simulink model "HVDC_Case_B"  (R2024b)
settings: Solver=VariableStepAuto  StartTime=0.0  StopTime=5  RelTol=1e-3
undefined symbols (not defined in the file): D11, Delta, leading, pulse
libraries: spsUniversalBridgeLib x4, spsSeriesRLCBranchLib x3, spsPLL3phLib x2, spsPower3phInstantaneousLib x2, spsPulseGeneratorThyristor12PulseLib x2, spsThreePhaseTransformerThreeWindingsLib x2, spsThreePhaseVIMeasurementLib x2, spsThreePhaseSourceLib x2, spsVoltageMeasurementLib x2, spsMeanLib x1, slpidlib x1, simulink x1
settings Model: Creator=Eng.Abd-Elrhman Saad  LastModifiedBy=Eng.Abd-Elrhman Saad

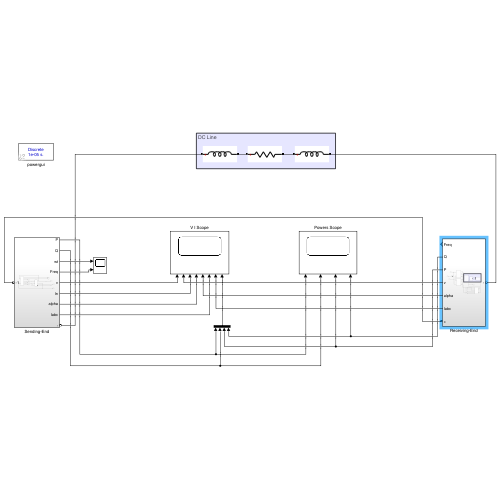
[thumbnail: Simulink's stored preview of the top-level diagram]
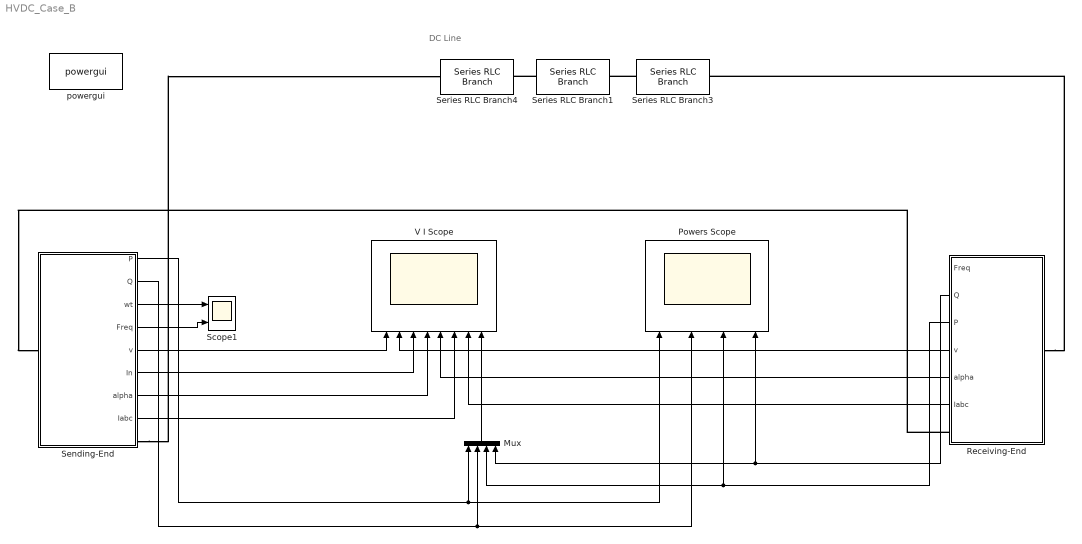
== system HVDC_Case_B ==
  note: DC Line
  Mux : Mux
  Powers Scope : Scope  NumInputPorts=4
  Receiving-End : Subsystem
  Scope1 : Scope  NumInputPorts=2
  Sending-End : Subsystem
  Series RLC Branch1 : spsSeriesRLCBranchLib/Series RLC Branch  LConnTagsString=__new0  RConnTagsString=__new0  BranchType=R  Resistance=5  Inductance=1e-3  SetiL0=off  InitialCurrent=0  Capacitance=1e-6  Setx0=off  InitialVoltage=0  Measurements=None
  Series RLC Branch3 : spsSeriesRLCBranchLib/Series RLC Branch  LConnTagsString=__new0  RConnTagsString=__new0  BranchType=L  Resistance=5  Inductance=0.3  SetiL0=off  InitialCurrent=1e5  Capacitance=1e-6  Setx0=off  InitialVoltage=0  Measurements=None
  Series RLC Branch4 : spsSeriesRLCBranchLib/Series RLC Branch  LConnTagsString=__new0  RConnTagsString=__new0  BranchType=L  Resistance=5  Inductance=0.3  SetiL0=off  InitialCurrent=1e5  Capacitance=1e-6  Setx0=off  InitialVoltage=0  Measurements=None
  V I Scope : Scope  NumInputPorts=8
  powergui : sps_lib/powergui  Priority=1  SimulationMode=Discrete  SampleTime=1e-5  frequency=60  Iterations=50  frequencyindice=50  Pbase=100e6  ErrMax=1e-4  UnitsV=kV  UnitsW=MW  buscounter=0  FunctionMessages=off  echomessages=off  EnableUseOfTLC=off  CurrentSourceSwitches=off  DisableSnubberDevices=off  DisableRonSwitches=off  DisableVfSwitches=off  DisplayEquations=off  AutomaticDiscreteSolvers=off  SolverType=Tustin/Backward Euler (TBE)  Interpol=off  ExternalGateDelay=off  methode=off  Ts=100  x0status=blocks  SPID=on  SwTol=0  HookPort=off  NonlinearTolerance=1e-4  nMaxIteration=100  ContinueOnMaxIteration=off  RestoreLinks=warning  ResistiveCurrentMeasurement=off  Frange=[0:2:500]  Ylog=off  Xlog=on  ShowGrid=off  save=off  variable=ZData  structure=0  ZoomFFT=off  StartTime=0.0  cycles=1  DisplayStyle=1  fundamental=60  FreqAxis=off  MaxFrequency=1000  frequencyindicesteady=1  RmsSteady=1  display=off
  wires:
  Mux/1 -> V I Scope/8
  Sending-End/2(Q) -> Powers Scope/2, Mux/2
  Sending-End/1(P) -> Mux/1, Powers Scope/1
  Sending-End/3(wt) -> Scope1/1
  Sending-End/4(Freq) -> Scope1/2
  Sending-End/5(v) -> V I Scope/1
  Sending-End/6(In) -> V I Scope/3
  Sending-End/7(alpha) -> V I Scope/4
  Sending-End/8(Iabc) -> V I Scope/6
  Receiving-End/2(Q) -> Mux/4, Powers Scope/4
  Receiving-End/3(P) -> Mux/3, Powers Scope/3
  Receiving-End/4(v) -> V I Scope/2
  Receiving-End/5(alpha) -> V I Scope/5
  Receiving-End/6(Iabc) -> V I Scope/7
  connections:
  Receiving-End/RConn1 -- Sending-End/LConn1
  Receiving-End/LConn1 -- Series RLC Branch3/RConn1
  Series RLC Branch1/LConn1 -- Series RLC Branch4/RConn1
  Sending-End/RConn1 -- Series RLC Branch4/LConn1
  Series RLC Branch3/LConn1 -- Series RLC Branch1/RConn1

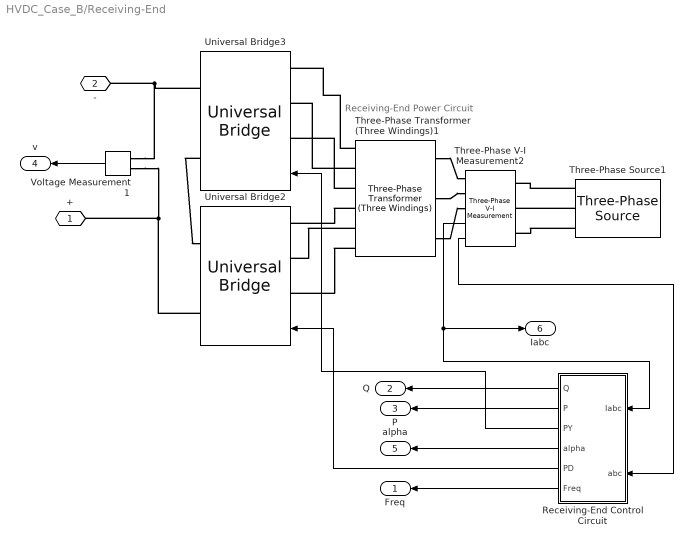
== system HVDC_Case_B/Receiving-End ==
  note: Receiving-End Power Circuit
  Receiving-End Control Circuit : Subsystem
  Three-Phase Transformer (Three Windings)1 : spsThreePhaseTransformerThreeWindingsLib/Three-Phase Transformer (Three Windings)  Winding1Connection=Yg  Winding2Connection=Delta (D11)  Winding3Connection=Y  CoreType=Three single-phase transformers  SetSaturation=off  Hysteresis=off  DataFile='hysteresis'  SetInitialFlux=off  Measurements=None  UNITS=pu  NominalPower=[ 2e9 , 50 ]  Winding1=[ 77.618e3 , 0.002 , 1e-6 ]  Winding2=[ 77.618e3 , 0.002 , 1e-6 ]  Winding3=[ 77.618e3 , 0.002 , 1e-6 ]  Rm=1e6  Lm=1e6  L0=1169.8  Saturation=[ 0,0 ; 0.0024,1.2 ; 1.0,1.52 ]  InitialFluxes=[1528.2 -1528.2 1337.2]  BreakLoop=off  DiscreteSolver=Trapezoidal iterative  DataType=off  TransfoNumber=1
      settings: LibrarySourceBlock=|
      | sps_lib/Power Grid Elements/Three-Phase
      | Transformer
      | (Three Windings)
  Three-Phase V-I Measurement2 : spsThreePhaseVIMeasurementLib/Three-Phase V-I Measurement  VoltageMeasurement=phase-to-ground  SetLabelV=off  LabelV=Vabc  Vpu=off  VpuLL=off  CurrentMeasurement=yes  SetLabelI=off  LabelI=Iabc  Ipu=off  Pbase=100e6  Vbase=500e3  OutputType=Complex  PhasorSimulation=off  PSBequivalent=0
  Three-Phase Source1 : spsThreePhaseSourceLib/Three-Phase Source  InternalConnection=Yg  VoltagePhases=off  Voltage=77.618e3  PhaseAngle=0  Voltage_phases=[25e3 25e3 25e3]/sqrt(3)  PhaseAngles_phases=[0 -120 +120]  Frequency=50  NonIdealSource=off  SpecifyImpedance=off  Resistance=0.8929  Inductance=16.58e-3  ShortCircuitLevel=100e6  BaseVoltage=25e3  XRratio=7  BusType=swing  Pref=10e3  Qref=0  Prefabc=[10e3, 10e3, 10e3]  Qrefabc=[0, 0, 0]  Qmin=-inf  Qmax=inf
  Universal Bridge2 : spsUniversalBridgeLib/Universal Bridge  Arms=3  SnubberResistance=1e5  SnubberCapacitance=inf  Device=Thyristors  Ron=1e-3  Lon=0  ForwardVoltages="[  0  0  ]"  ForwardVoltage=0  GTOparameters=[ 10e-6 , 20e-6 ]  IGBTparameters=[ 1e-6 , 2e-6 ]  Measurements=None  Measurements_2=None  converterType=Rectifier
  Universal Bridge3 : spsUniversalBridgeLib/Universal Bridge  Arms=3  SnubberResistance=1e5  SnubberCapacitance=inf  Device=Thyristors  Ron=1e-3  Lon=0  ForwardVoltages="[  0  0  ]"  ForwardVoltage=0  GTOparameters=[ 10e-6 , 20e-6 ]  IGBTparameters=[ 1e-6 , 2e-6 ]  Measurements=None  Measurements_2=None  converterType=Rectifier
  Voltage Measurement1 : spsVoltageMeasurementLib/Voltage Measurement  PhasorSimulation=off  OutputType=Complex  PSBequivalent=0
  + : PMIOPort  Side=Right
  - : PMIOPort  Port=2  Side=Left
  Freq : Outport
  Q : Outport  Port=2
  P : Outport  Port=3
  v : Outport  Port=4
  alpha : Outport  Port=5
  Iabc : Outport  Port=6
  wires:
  Receiving-End Control Circuit/3(PY) -> Universal Bridge3/1
  Receiving-End Control Circuit/5(PD) -> Universal Bridge2/1
  Three-Phase V-I Measurement2/1 -> Receiving-End Control Circuit/2(abc)
  Three-Phase V-I Measurement2/2 -> Receiving-End Control Circuit/1(Iabc), Iabc/1
  Receiving-End Control Circuit/2(P) -> P/1
  Receiving-End Control Circuit/1(Q) -> Q/1
  Voltage Measurement1/1 -> v/1
  Receiving-End Control Circuit/4(alpha) -> alpha/1
  Receiving-End Control Circuit/6(Freq) -> Freq/1
  connections:
  Voltage Measurement1/LConn1 -- -/RConn1 -- Universal Bridge3/RConn2
  Universal Bridge3/RConn1 -- Universal Bridge2/RConn2
  Voltage Measurement1/LConn2 -- Universal Bridge2/RConn1 -- +/RConn1
  Three-Phase Transformer (Three Windings)1/LConn1 -- Three-Phase V-I Measurement2/RConn1
  Three-Phase Source1/RConn3 -- Three-Phase V-I Measurement2/LConn3
  Three-Phase Source1/RConn2 -- Three-Phase V-I Measurement2/LConn2
  Three-Phase Source1/RConn1 -- Three-Phase V-I Measurement2/LConn1
  Three-Phase Transformer (Three Windings)1/LConn2 -- Three-Phase V-I Measurement2/RConn2
  Three-Phase Transformer (Three Windings)1/LConn3 -- Three-Phase V-I Measurement2/RConn3
  Three-Phase Transformer (Three Windings)1/RConn1 -- Universal Bridge2/LConn1
  Three-Phase Transformer (Three Windings)1/RConn2 -- Universal Bridge2/LConn2
  Three-Phase Transformer (Three Windings)1/RConn3 -- Universal Bridge2/LConn3
  Three-Phase Transformer (Three Windings)1/RConn4 -- Universal Bridge3/LConn1
  Three-Phase Transformer (Three Windings)1/RConn5 -- Universal Bridge3/LConn2
  Three-Phase Transformer (Three Windings)1/RConn6 -- Universal Bridge3/LConn3

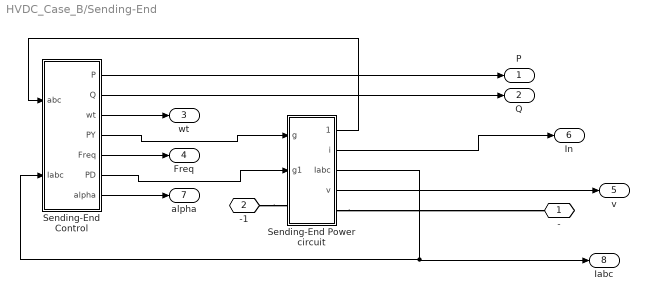
== system HVDC_Case_B/Sending-End ==
  Sending-End Control : Subsystem
  Sending-End Power circuit : Subsystem
  - : PMIOPort  Side=Right
  -1 : PMIOPort  Port=2  Side=Left
  P : Outport
  Q : Outport  Port=2
  wt : Outport  Port=3
  Freq : Outport  Port=4
  v : Outport  Port=5
  In : Outport  Port=6
  alpha : Outport  Port=7
  Iabc : Outport  Port=8
  wires:
  Sending-End Power circuit/3(Iabc) -> Iabc/1, Sending-End Control/2(Iabc)
  Sending-End Power circuit/1(Vabc) -> Sending-End Control/1(abc)
  Sending-End Power circuit/2(i) -> In/1
  Sending-End Control/6(PD) -> Sending-End Power circuit/2(g1)
  Sending-End Control/4(PY) -> Sending-End Power circuit/1(g)
  Sending-End Control/2(Q) -> Q/1
  Sending-End Power circuit/4(v) -> v/1
  Sending-End Control/5(Freq) -> Freq/1
  Sending-End Control/7(alpha) -> alpha/1
  Sending-End Control/3(wt) -> wt/1
  Sending-End Control/1(P) -> P/1
  connections:
  -1/RConn1 -- Sending-End Power circuit/LConn1
  Sending-End Power circuit/RConn1 -- -/RConn1

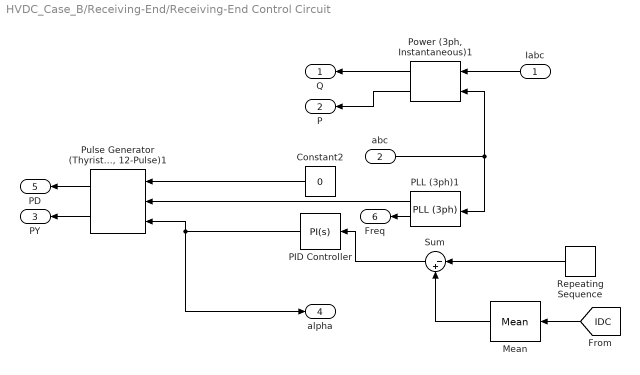
== system HVDC_Case_B/Receiving-End/Receiving-End Control Circuit ==
  Iabc : Inport
  abc : Inport  Port=2
  Constant2 : Constant  Value=0
  Mean : spsMeanLib/Mean  Freq=50  Vinit=0  Ts=0
  PID Controller : slpidlib/PID Controller  Controller=PI  Form=Parallel  TimeDomain=Continuous-time  UseExternalTs=off  SampleTime=-1  IntegratorMethod=Forward Euler  FilterMethod=Forward Euler  ControllerParametersSource=internal  P=0.003  I=0.05  UseKiTs=off  D=0  UseExternalDerivativeSource=off  N=100  UseFilter=on  TunerSelectOption=Transfer Function Based (PID Tuner App)  InitialConditionSource=internal  InitialConditionForIntegrator=110  InitialConditionForFilter=0  DifferentiatorICPrevScaledInput=0  ExternalReset=none  TrackingMode=off  Kt=1  LimitOutput=on  SatLimitsSource=internal  UpperSaturationLimit=160  LowerSaturationLimit=100  LinearizeAsGain=on  AntiWindupMode=none  Kb=1  LimitIntegrator=off  UpperIntegratorSaturationLimit=inf  LowerIntegratorSaturationLimit=-inf  POutMin=[]  POutMax=[]  IOutMin=[]  IOutMax=[]  DOutMin=[]  DOutMax=[]  NOutMin=[]  NOutMax=[]  SumOutMin=[]  SumOutMax=[]  SaturationOutMin=[]  SaturationOutMax=[]  PParamMin=[]  PParamMax=[]  IParamMin=[]  IParamMax=[]  DParamMin=[]  DParamMax=[]  NParamMin=[]  NParamMax=[]  KbParamMin=[]  KbParamMax=[]  KtParamMin=[]  KtParamMax=[]  KbOutMin=[]  KbOutMax=[]  KtOutMin=[]  KtOutMax=[]  IntegratorOutMin=[]  IntegratorOutMax=[]  FilterOutMin=[]  FilterOutMax=[]  SumI1OutMin=[]  SumI1OutMax=[]  SumI2OutMin=[]  SumI2OutMax=[]  SumI3OutMin=[]  SumI3OutMax=[]  SumI4OutMin=[]  SumI4OutMax=[]  SumDOutMin=[]  SumDOutMax=[]  DifferentiatorOutMin=[]  DifferentiatorOutMax=[]  FilterDiffOutCoefMin=[]  FilterDiffOutCoefMax=[]  ReciprocalOutMin=[]  ReciprocalOutMax=[]  SumDenOutMin=[]  SumDenOutMax=[]  SumNumOutMin=[]  SumNumOutMax=[]  DivideOutMin=[]  DivideOutMax=[]  UdiffTsProdOutMin=[]  UdiffTsProdOutMax=[]  NTsProdOutMin=[]  NTsProdOutMax=[]  UintegralTsProdOutMin=[]  UintegralTsProdOutMax=[]  UngainTsProdOutMin=[]  UngainTsProdOutMax=[]  ClampingZeroOutDataTypeStr=Inherit: Inherit via back propagation  ClampingZeroOutMin=[]  ClampingZeroOutMax=[]  FilterDenConstantOutDataTypeStr=Inherit: Inherit via back propagation  FilterDenConstantOutMin=[]  FilterDenConstantOutMax=[]  PCopyOutDataTypeStr=Inherit: Inherit via back propagation  PCopyOutMin=[]  PCopyOutMax=[]  NCopyOutDataTypeStr=Inherit: Inherit via back propagation  NCopyOutMin=[]  NCopyOutMax=[]  IntegratorContinuousStateAttributes=''  IntegratorStateMustResolveToSignalObject=off  IntegratorRTWStateStorageClass=Auto  FilterContinuousStateAttributes=''  FilterStateMustResolveToSignalObject=off  FilterRTWStateStorageClass=Auto  ParallelPVariant=InternalParameters  IdealPVariant=Disabled  IVariant=InternalParameters  DVariant=Disabled  IntegratorVariant=Continuous  SatVariant=Enabled  AWVariant=Passthrough  PCopyVariant=Disabled  TRVariant=Disabled  FdbkBlocksVariant=Forward  IdealPFdbkVariant=Disabled  SatFdbkVariant=Disabled  DerivativeFilterVariant=Disabled  NVariant=Disabled  NCopyVariant=Disabled_SignalSpec  FilterICVariant=Disabled  IntegratorICVariant=InternalICs  ExternalResetVariant=Disabled  TRSumVariant=Passthrough  SumFdbkVariant=Disabled  SumVariant=Sum_PI  TsampFilterVariant=InternalTs  TsampNgainVariant=Passthrough  TsampIntegralVariant=Disabled_SignalSpec  ExternalSaturationOutDataTypeStr=Inherit: Same as second input  DerivativeSourceVariant=Disabled  PreIntVariant=InternalPreInt
  PLL (3ph)1 : spsPLL3phLib/PLL (3ph)  Fmin=45  Par_Init=[0, 50]  ParK=[180, 3200, 1]  TcD=1e-4  MaxRateChangeFreq=12  FilterCutOffFreq=25  Ts=0  AGC=on
  "Power (3ph, Instantaneous)1" : spsPower3phInstantaneousLib/Power (3ph, Instantaneous)
  "Pulse Generator (Thyristor, 12-Pulse)1" : spsPulseGeneratorThyristor12PulseLib/Pulse Generator (Thyristor, 12-Pulse)  GenType=12-pulse  Delta=D11 (leading)  pwidth=30  Double_Pulse=off  Ts=0
      settings: LibrarySourceBlock=|
      | sps_lib/Power Electronics/Power Electronics Control/Pulse Generator
      | (Thyristor, 12-Pulse)
  Repeating Sequence : simulink/Sources/Repeating Sequence  rep_seq_t=[0, 0.2, 2, 2.0001, 4, 4.0001, 10]  rep_seq_y=[0, 6650, 6650, 5700, 5700, 6650, 6650]
  Sum : Sum  Inputs=|-+
  Q : Outport
  P : Outport  Port=2
  PY : Outport  Port=3
  alpha : Outport  Port=4
  PD : Outport  Port=5
  Freq : Outport  Port=6
  wires:
  Constant2/1 -> "Pulse Generator (Thyristor, 12-Pulse)1"/3
  abc/1 -> "Power (3ph, Instantaneous)1"/1, PLL (3ph)1/1
  PLL (3ph)1/2 -> "Pulse Generator (Thyristor, 12-Pulse)1"/2
  "Power (3ph, Instantaneous)1"/2 -> Q/1
  PID Controller/1 -> alpha/1, "Pulse Generator (Thyristor, 12-Pulse)1"/1
  "Pulse Generator (Thyristor, 12-Pulse)1"/2 -> PD/1
  PLL (3ph)1/1 -> Freq/1
  "Pulse Generator (Thyristor, 12-Pulse)1"/1 -> PY/1
  Iabc/1 -> "Power (3ph, Instantaneous)1"/2
  "Power (3ph, Instantaneous)1"/1 -> P/1
  Sum/1 -> PID Controller/1
  Mean/1 -> Sum/2
  Repeating Sequence/1 -> Sum/1
  [IDC] -> Mean/1

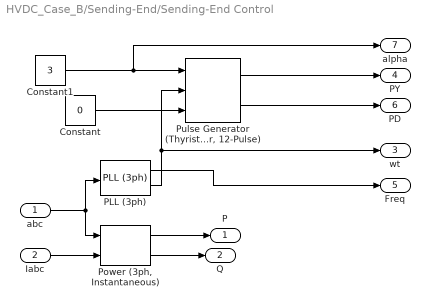
== system HVDC_Case_B/Sending-End/Sending-End Control ==
  abc : Inport
  Iabc : Inport  Port=2
  Constant : Constant  Value=0
  Constant1 : Constant  Value=3
  PLL (3ph) : spsPLL3phLib/PLL (3ph)  Fmin=45  Par_Init=[0, 50]  ParK=[180, 3200, 1]  TcD=1e-4  MaxRateChangeFreq=12  FilterCutOffFreq=25  Ts=0  AGC=on
  "Power (3ph, Instantaneous)" : spsPower3phInstantaneousLib/Power (3ph, Instantaneous)
  "Pulse Generator (Thyristor, 12-Pulse)" : spsPulseGeneratorThyristor12PulseLib/Pulse Generator (Thyristor, 12-Pulse)  GenType=12-pulse  Delta=D11 (leading)  pwidth=30  Double_Pulse=off  Ts=0
      settings: LibrarySourceBlock=|
      | sps_lib/Power Electronics/Power Electronics Control/Pulse Generator
      | (Thyristor, 12-Pulse)
  P : Outport
  Q : Outport  Port=2
  wt : Outport  Port=3
  PY : Outport  Port=4
  Freq : Outport  Port=5
  PD : Outport  Port=6
  alpha : Outport  Port=7
  wires:
  PLL (3ph)/2 -> "Pulse Generator (Thyristor, 12-Pulse)"/2, wt/1
  Constant1/1 -> alpha/1, "Pulse Generator (Thyristor, 12-Pulse)"/1
  Iabc/1 -> "Power (3ph, Instantaneous)"/2
  Constant/1 -> "Pulse Generator (Thyristor, 12-Pulse)"/3
  abc/1 -> "Power (3ph, Instantaneous)"/1, PLL (3ph)/1
  "Power (3ph, Instantaneous)"/1 -> P/1
  "Pulse Generator (Thyristor, 12-Pulse)"/2 -> PD/1
  "Power (3ph, Instantaneous)"/2 -> Q/1
  "Pulse Generator (Thyristor, 12-Pulse)"/1 -> PY/1
  PLL (3ph)/1 -> Freq/1

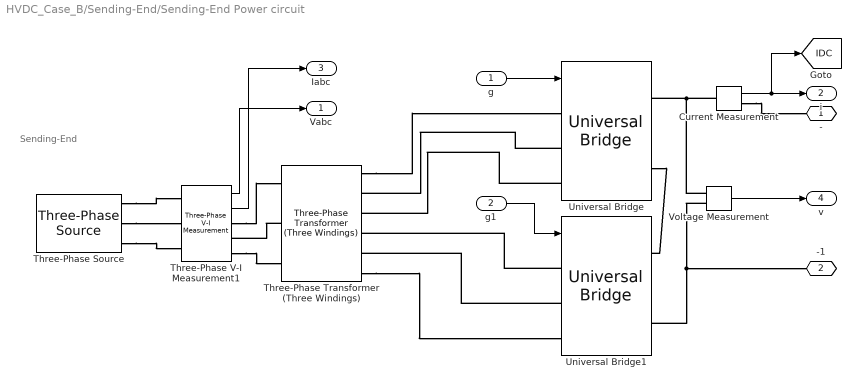
== system HVDC_Case_B/Sending-End/Sending-End Power circuit ==
  note: Sending-End
  g : Inport
  g1 : Inport  Port=2
  Current Measurement : spsCurrentMeasurementLib/Current Measurement  PhasorSimulation=off  OutputType=Complex  PSBequivalent=0
  Three-Phase Transformer (Three Windings) : spsThreePhaseTransformerThreeWindingsLib/Three-Phase Transformer (Three Windings)  Winding1Connection=Yg  Winding2Connection=Y  Winding3Connection=Delta (D11)  CoreType=Three single-phase transformers  SetSaturation=off  Hysteresis=off  DataFile='hysteresis'  SetInitialFlux=off  Measurements=None  UNITS=pu  NominalPower=[ 2e9 , 50 ]  Winding1=[56.3925e3 , 0.0002 , 1e-6]  Winding2=[56.3925e3 , 0.0002 , 1e-6]  Winding3=[56.3925e3 , 0.0002 , 1e-6]  Rm=1e6  Lm=1e6  L0=1169.8  Saturation=[ 0,0 ; 0.0024,1.2 ; 1.0,1.52 ]  InitialFluxes=[1528.2 -1528.2 1337.2]  BreakLoop=off  DiscreteSolver=Trapezoidal iterative  DataType=off  TransfoNumber=1
      settings: LibrarySourceBlock=|
      | sps_lib/Power Grid Elements/Three-Phase
      | Transformer
      | (Three Windings)
  Three-Phase V-I Measurement1 : spsThreePhaseVIMeasurementLib/Three-Phase V-I Measurement  VoltageMeasurement=phase-to-ground  SetLabelV=off  LabelV=Vabc  Vpu=off  VpuLL=off  CurrentMeasurement=yes  SetLabelI=off  LabelI=Iabc  Ipu=off  Pbase=100e6  Vbase=500e3  OutputType=Complex  PhasorSimulation=off  PSBequivalent=0
  Three-Phase Source : spsThreePhaseSourceLib/Three-Phase Source  InternalConnection=Yg  VoltagePhases=off  Voltage=56.3925e3  PhaseAngle=0  Voltage_phases=[25e3 25e3 25e3]/sqrt(3)  PhaseAngles_phases=[0 -120 +120]  Frequency=50  NonIdealSource=off  SpecifyImpedance=off  Resistance=0.8929  Inductance=16.58e-3  ShortCircuitLevel=100e6  BaseVoltage=25e3  XRratio=7  BusType=swing  Pref=10e3  Qref=0  Prefabc=[10e3, 10e3, 10e3]  Qrefabc=[0, 0, 0]  Qmin=-inf  Qmax=inf
  Universal Bridge : spsUniversalBridgeLib/Universal Bridge  Arms=3  SnubberResistance=1e5  SnubberCapacitance=inf  Device=Thyristors  Ron=1e-3  Lon=0  ForwardVoltages="[  0  0  ]"  ForwardVoltage=0  GTOparameters=[ 10e-6 , 20e-6 ]  IGBTparameters=[ 1e-6 , 2e-6 ]  Measurements=None  Measurements_2=None  converterType=Rectifier
  Universal Bridge1 : spsUniversalBridgeLib/Universal Bridge  Arms=3  SnubberResistance=1e5  SnubberCapacitance=inf  Device=Thyristors  Ron=1e-3  Lon=0  ForwardVoltages="[  0  0  ]"  ForwardVoltage=0  GTOparameters=[ 10e-6 , 20e-6 ]  IGBTparameters=[ 1e-6 , 2e-6 ]  Measurements=None  Measurements_2=None  converterType=Rectifier
  Voltage Measurement : spsVoltageMeasurementLib/Voltage Measurement  PhasorSimulation=off  OutputType=Complex  PSBequivalent=0
  - : PMIOPort  Side=Right
  -1 : PMIOPort  Port=2  Side=Left
  Vabc : Outport
  i : Outport  Port=2
  Iabc : Outport  Port=3
  v : Outport  Port=4
  tag scope: IDC=global
  wires:
  g/1 -> Universal Bridge/1
  Three-Phase V-I Measurement1/1 -> Vabc/1
  Three-Phase V-I Measurement1/2 -> Iabc/1
  Current Measurement/1 -> [IDC], i/1
  Voltage Measurement/1 -> v/1
  g1/1 -> Universal Bridge1/1
  connections:
  Three-Phase Transformer (Three Windings)/RConn1 -- Universal Bridge/LConn1
  Current Measurement/LConn1 -- Universal Bridge/RConn1 -- Voltage Measurement/LConn1
  Three-Phase Transformer (Three Windings)/RConn6 -- Universal Bridge1/LConn3
  Voltage Measurement/LConn2 -- Universal Bridge1/RConn2 -- -1/RConn1
  Universal Bridge/RConn2 -- Universal Bridge1/RConn1
  Current Measurement/RConn1 -- -/RConn1
  Universal Bridge/LConn2 -- Three-Phase Transformer (Three Windings)/RConn2
  Universal Bridge1/LConn1 -- Three-Phase Transformer (Three Windings)/RConn4
  Universal Bridge1/LConn2 -- Three-Phase Transformer (Three Windings)/RConn5
  Three-Phase Source/RConn2 -- Three-Phase V-I Measurement1/LConn2
  Three-Phase Source/RConn3 -- Three-Phase V-I Measurement1/LConn3
  Three-Phase V-I Measurement1/RConn3 -- Three-Phase Transformer (Three Windings)/LConn3
  Three-Phase Source/RConn1 -- Three-Phase V-I Measurement1/LConn1
  Three-Phase Transformer (Three Windings)/LConn2 -- Three-Phase V-I Measurement1/RConn2
  Three-Phase V-I Measurement1/RConn1 -- Three-Phase Transformer (Three Windings)/LConn1
  Universal Bridge/LConn3 -- Three-Phase Transformer (Three Windings)/RConn3
